simulink model "Transformations"  (R2020b)
settings: Solver=FixedStepAuto  StartTime=0.0  StopTime=0.1  FixedStep=5e-6  RelTol=1e-3  EnableMultiTasking=on
settings Model: Creator=Lei  LastModifiedBy=Ray
settings DataIOCC: LimitDataPoints=on  SaveFormat=Array  ReturnWorkspaceOutputs=off
settings OptimizationCC: LifeSpan=inf
settings DebuggingCC: SolverPrmCheckMsg=warning  SFUnexpectedBacktrackingDiag=warning  SFNoUnconditionalDefaultTransitionDiag=warning  SFExecutionAtInitializationDiag=none  ArithmeticOperatorsInVariantConditions=warning
settings HardwareCC: ProdBitPerPointer=32  ProdBitPerSizeT=32  ProdBitPerPtrDiffT=32  ProdLargestAtomicFloat=None  ProdIntDivRoundTo=Undefined  ProdEndianess=Unspecified  ProdWordSize=32  ProdHWDeviceType=32-bit Generic
settings ModelReferenceCC: PropagateSignalLabelsOutOfModel=off
settings SFSimCC: SimUseLocalCustomCode=off  CustomCodeUndefinedFunction=UseInterfaceOnly
settings RTWCC: RTWUseLocalCustomCode=off
settings CodeAppCC: StateflowObjectComments=on
settings GRTTargetCC: TargetLangStandard=C89/C90 (ANSI)
settings ConfigComp: CovMetricSettings=dw  CovSaveCumulativeToWorkspaceVar=on  CovSaveSingleToWorkspaceVar=on  CovExternalEMLEnable=off  CovSFcnEnable=off

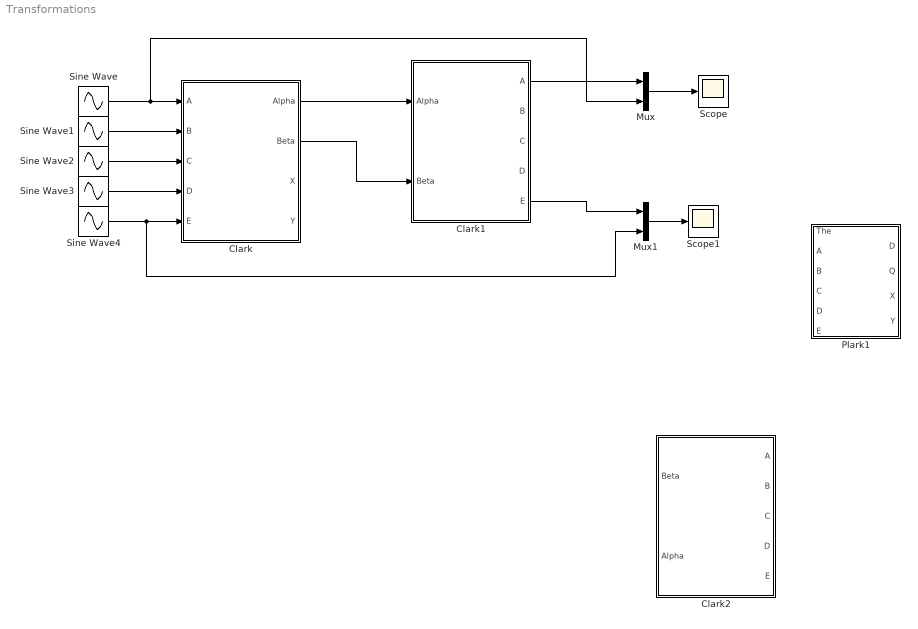
== system Transformations ==
  Clark : Subsystem
  Clark1 : Subsystem
  Clark2 : Subsystem
  Mux : Mux  Inputs=2
  Mux1 : Mux  Inputs=2
  Plark1 : Subsystem
  Scope : Scope
  Scope1 : Scope
  Sine Wave : Sin  Amplitude=100  Frequency=2*pi*50  SampleTime=0
  Sine Wave1 : Sin  Amplitude=100  Frequency=2*pi*50  Phase=-2*pi/5  SampleTime=0
  Sine Wave2 : Sin  Amplitude=100  Frequency=2*pi*50  Phase=-4*pi/5  SampleTime=0
  Sine Wave3 : Sin  Amplitude=100  Frequency=2*pi*50  Phase=-6*pi/5  SampleTime=0
  Sine Wave4 : Sin  Amplitude=100  Frequency=2*pi*50  Phase=-8*pi/5  SampleTime=0
  wires:
  Sine Wave/1 -> Mux/2, Clark/1(A)
  Sine Wave1/1 -> Clark/2(B)
  Sine Wave2/1 -> Clark/3(C)
  Sine Wave3/1 -> Clark/4(D)
  Sine Wave4/1 -> Mux1/2, Clark/5(E)
  Clark/1(Alpha) -> Clark1/1(Alpha)
  Clark/2(Beta) -> Clark1/2(Beta)
  Clark1/1(A) -> Mux/1
  Mux/1 -> Scope/1
  Clark1/5(E) -> Mux1/1
  Mux1/1 -> Scope1/1

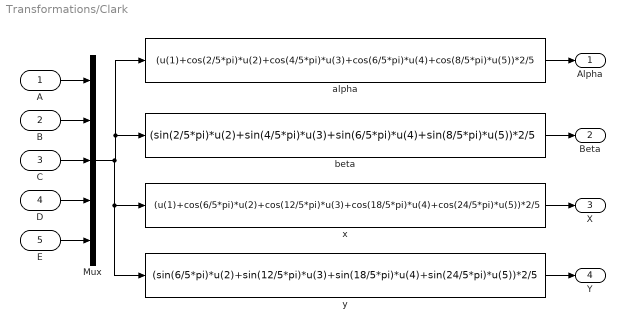
== system Transformations/Clark ==
  A : Inport
  B : Inport  Port=2
  C : Inport  Port=3
  D : Inport  Port=4
  E : Inport  Port=5
  Mux : Mux  Inputs=5
  alpha : Fcn  Expr=(u(1)+cos(2/5*pi)*u(2)+cos(4/5*pi)*u(3)+cos(6/5*pi)*u(4)+cos(8/5*pi)*u(5))*2/5
  beta : Fcn  Expr=(sin(2/5*pi)*u(2)+sin(4/5*pi)*u(3)+sin(6/5*pi)*u(4)+sin(8/5*pi)*u(5))*2/5
  "x " : Fcn  Expr=(u(1)+cos(6/5*pi)*u(2)+cos(12/5*pi)*u(3)+cos(18/5*pi)*u(4)+cos(24/5*pi)*u(5))*2/5
  "y " : Fcn  Expr=(sin(6/5*pi)*u(2)+sin(12/5*pi)*u(3)+sin(18/5*pi)*u(4)+sin(24/5*pi)*u(5))*2/5
  Alpha : Outport
  Beta : Outport  Port=2
  X : Outport  Port=3
  Y : Outport  Port=4
  wires:
  alpha/1 -> Alpha/1
  B/1 -> Mux/2
  C/1 -> Mux/3
  A/1 -> Mux/1
  beta/1 -> Beta/1
  D/1 -> Mux/4
  E/1 -> Mux/5
  Mux/1 -> "x "/1, "y "/1, alpha/1, beta/1
  "x "/1 -> X/1
  "y "/1 -> Y/1

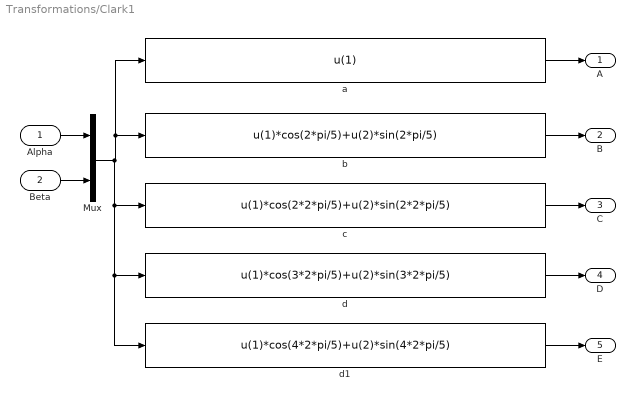
== system Transformations/Clark1 ==
  Alpha : Inport
  Beta : Inport  Port=2
  Mux : Mux  Inputs=2
  a : Fcn  Expr=u(1)
  b : Fcn  Expr=u(1)*cos(2*pi/5)+u(2)*sin(2*pi/5)
  c : Fcn  Expr=u(1)*cos(2*2*pi/5)+u(2)*sin(2*2*pi/5)
  d : Fcn  Expr=u(1)*cos(3*2*pi/5)+u(2)*sin(3*2*pi/5)
  d1 : Fcn  Expr=u(1)*cos(4*2*pi/5)+u(2)*sin(4*2*pi/5)
  A : Outport
  B : Outport  Port=2
  C : Outport  Port=3
  D : Outport  Port=4
  E : Outport  Port=5
  wires:
  Mux/1 -> d1/1, d/1, c/1, b/1, a/1
  Alpha/1 -> Mux/1
  Beta/1 -> Mux/2
  a/1 -> A/1
  b/1 -> B/1
  c/1 -> C/1
  d/1 -> D/1
  d1/1 -> E/1

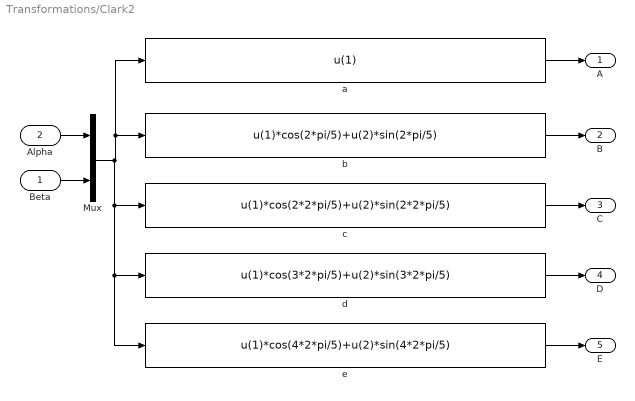
== system Transformations/Clark2 ==
  Beta : Inport
  Alpha : Inport  Port=2
  Mux : Mux  Inputs=2
  a : Fcn  Expr=u(1)
  b : Fcn  Expr=u(1)*cos(2*pi/5)+u(2)*sin(2*pi/5)
  c : Fcn  Expr=u(1)*cos(2*2*pi/5)+u(2)*sin(2*2*pi/5)
  d : Fcn  Expr=u(1)*cos(3*2*pi/5)+u(2)*sin(3*2*pi/5)
  e : Fcn  Expr=u(1)*cos(4*2*pi/5)+u(2)*sin(4*2*pi/5)
  A : Outport
  B : Outport  Port=2
  C : Outport  Port=3
  D : Outport  Port=4
  E : Outport  Port=5
  wires:
  Mux/1 -> e/1, d/1, c/1, b/1, a/1
  Alpha/1 -> Mux/1
  Beta/1 -> Mux/2
  a/1 -> A/1
  b/1 -> B/1
  c/1 -> C/1
  d/1 -> D/1
  e/1 -> E/1

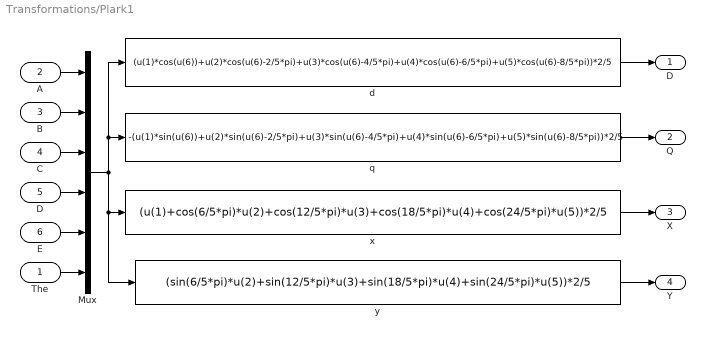
== system Transformations/Plark1 ==
  The : Inport
  A : Inport  Port=2
  B : Inport  Port=3
  C : Inport  Port=4
  D : Inport  Port=5
  E : Inport  Port=6
  Mux : Mux  Inputs=6
  d : Fcn  Expr=(u(1)*cos(u(6))+u(2)*cos(u(6)-2/5*pi)+u(3)*cos(u(6)-4/5*pi)+u(4)*cos(u(6)-6/5*pi)+u(5)*cos(u(6)-8/5*pi))*2/5
  q : Fcn  Expr=-(u(1)*sin(u(6))+u(2)*sin(u(6)-2/5*pi)+u(3)*sin(u(6)-4/5*pi)+u(4)*sin(u(6)-6/5*pi)+u(5)*sin(u(6)-8/5*pi))*2/5
  "x " : Fcn  Expr=(u(1)+cos(6/5*pi)*u(2)+cos(12/5*pi)*u(3)+cos(18/5*pi)*u(4)+cos(24/5*pi)*u(5))*2/5
  "y " : Fcn  Expr=(sin(6/5*pi)*u(2)+sin(12/5*pi)*u(3)+sin(18/5*pi)*u(4)+sin(24/5*pi)*u(5))*2/5
  "D " : Outport
  Q : Outport  Port=2
  X : Outport  Port=3
  Y : Outport  Port=4
  wires:
  d/1 -> "D "/1
  B/1 -> Mux/2
  C/1 -> Mux/3
  A/1 -> Mux/1
  D/1 -> Mux/4
  E/1 -> Mux/5
  The/1 -> Mux/6
  Mux/1 -> q/1, d/1, "y "/1, "x "/1
  q/1 -> Q/1
  "x "/1 -> X/1
  "y "/1 -> Y/1
